simulink model "kinovaMicoSimscapeModel"  (R2021b)
settings: Solver=VariableStepAuto  StartTime=0.0  StopTime=0.3  FixedStep=0.01  RelTol=1e-3
PostLoadFcn:
  | micoRigidBodyTreeCreation;
  | IC=deg2rad([-90,180,180,0,0,0]);
  | interactiveHomePosition=deg2rad([-90 90 177.5 90 0 0]');
  | load("./KinovaMicoSimscapeVariantConfigurations.mat");
values from neighbouring files (symbols this model uses):
  micoCandlePosition = deg2rad([0,180,180,0,0,0])    [KinovaMicoSimscapeInitializeScript.m]    (also in generatingRandomTrajectory.m)
  ViaPointsTaskSpace = [ViaPointsTaskSpace;[[pi;0;pi],[pi;0;pi],[pi;0;pi],[pi;0;pi],[0;0;0],[0;0;0],[pi;0;pi]]]    [KinovaMicoSimscapeInitializeScript.m]    (also in generatingRandomTrajectory.m = [ViaPointsTaskSpace;zeros(3,7)])
undefined symbols (not defined in the file or in its folder): Mico, ViaPointsJointSpace, X, Y, Z
libraries: sm_lib x26, nesl_utility x19, robotcorelib x4, robotmaniplib x3, pid_lib x2
(part 29 of 50)

== matlab function kinovaMicoSimscapeModel/Variant Subsystem/TaskSpaceController/Adaptive PID/VectorManipulation ==
  data: dqr output; ddqr output; S output; q input; dq input; qd input; dqd input; ddqd input
function [dqr,ddqr,S] = VectorManipulation(q,dq,qd,dqd,ddqd)
%% Unpacking the measurements/desired points
%Unpackage the incoming reference/measured states

q1 = q(1);
q2 = q(2);
q3 = q(3);
q4 = q(4);
q5 = q(5);
q6 = q(6);

dq1 = dq(1);
dq2 = dq(2);
dq3 = dq(3);
dq4 = dq(4);
dq5 = dq(5);
dq6 = dq(6);

qd1 = qd(1);
qd2 = qd(2);
qd3 = qd(3);
qd4 = qd(4);
qd5 = qd(5);
qd6 = qd(6);

dqd1 = dqd(1);
dqd2 = dqd(2);
dqd3 = dqd(3);
dqd4 = dqd(4);
dqd5 = dqd(5);
dqd6 = dqd(6);

ddqd1 = ddqd(1);
ddqd2 = ddqd(2);
ddqd3 = ddqd(3);
ddqd4 = ddqd(4);
ddqd5 = ddqd(5);
ddqd6 = ddqd(6);

qError=q-qd;
dqError=dq-dqd;

%Define parameters
lambda=10*eye(6);
K=10;

dqr=dqd-lambda*qError;
ddqr=ddqd-lambda*dqError;

dqr1=dqr(1);
dqr2=dqr(2);
dqr3=dqr(3);
dqr4=dqr(4);
dqr5=dqr(5);
dqr6=dqr(6);

ddqr1=ddqr(1);
ddqr2=ddqr(2);
ddqr3=ddqr(3);
ddqr4=ddqr(4);
ddqr5=ddqr(5);
ddqr6=ddqr(6);

S=dqError+lambda*qError;

== matlab function kinovaMicoSimscapeModel/Variant Subsystem/TaskSpaceController/Enabled Subsystem/G_RNE ==
  data: q input; G output
function G = fcn(q)

q1 = q(1);
q2 = q(2);
q3 = q(3);
q4 = q(4);
q5 = q(5);
q6 = q(6);


G1 = 0;
 
G2 = (1116181*sin(q2))/2000000 + (41927301*cos(q2)*sin(q3))/200000000 - (41927301*cos(q3)*sin(q2))/200000000 + (164391*sin(q2)*sin(q3)*sin(q4))/5000000 + (164391*cos(q2)*cos(q3)*sin(q4))/5000000 + (213189*cos(q2)*cos(q5)*sin(q3))/200000000 - (213189*cos(q3)*cos(q5)*sin(q2))/200000000 + (3038029*3^(1/2)*cos(q2)*cos(q3)*sin(q4))/200000000 + (85507*3^(1/2)*cos(q2)*cos(q5)*sin(q3))/10000000 - (85507*3^(1/2)*cos(q3)*cos(q5)*sin(q2))/10000000 + (3038029*3^(1/2)*sin(q2)*sin(q3)*sin(q4))/200000000 - (85507*cos(q2)*cos(q3)*cos(q4)*sin(q5))/5000000 - (85507*cos(q2)*cos(q3)*cos(q5)*sin(q4))/10000000 - (85507*cos(q4)*sin(q2)*sin(q3)*sin(q5))/5000000 - (85507*cos(q5)*sin(q2)*sin(q3)*sin(q4))/10000000 - (71063*3^(1/2)*cos(q2)*cos(q3)*cos(q4)*sin(q5))/100000000 - (71063*3^(1/2)*cos(q2)*cos(q3)*cos(q5)*sin(q4))/200000000 - (71063*3^(1/2)*cos(q4)*sin(q2)*sin(q3)*sin(q5))/100000000 - (71063*3^(1/2)*cos(q5)*sin(q2)*sin(q3)*sin(q4))/200000000;
 
G3 = (41927301*cos(q3)*sin(q2))/200000000 - (41927301*cos(q2)*sin(q3))/200000000 - (164391*sin(q2)*sin(q3)*sin(q4))/5000000 - (164391*cos(q2)*cos(q3)*sin(q4))/5000000 - (213189*cos(q2)*cos(q5)*sin(q3))/200000000 + (213189*cos(q3)*cos(q5)*sin(q2))/200000000 - (3038029*3^(1/2)*cos(q2)*cos(q3)*sin(q4))/200000000 - (85507*3^(1/2)*cos(q2)*cos(q5)*sin(q3))/10000000 + (85507*3^(1/2)*cos(q3)*cos(q5)*sin(q2))/10000000 - (3038029*3^(1/2)*sin(q2)*sin(q3)*sin(q4))/200000000 + (85507*cos(q2)*cos(q3)*cos(q4)*sin(q5))/5000000 + (85507*cos(q2)*cos(q3)*cos(q5)*sin(q4))/10000000 + (85507*cos(q4)*sin(q2)*sin(q3)*sin(q5))/5000000 + (85507*cos(q5)*sin(q2)*sin(q3)*sin(q4))/10000000 + (71063*3^(1/2)*cos(q2)*cos(q3)*cos(q4)*sin(q5))/100000000 + (71063*3^(1/2)*cos(q2)*cos(q3)*cos(q5)*sin(q4))/200000000 + (71063*3^(1/2)*cos(q4)*sin(q2)*sin(q3)*sin(q5))/100000000 + (71063*3^(1/2)*cos(q5)*sin(q2)*sin(q3)*sin(q4))/200000000;
 
G4 = (164391*cos(q3)*cos(q4)*sin(q2))/5000000 - (164391*cos(q2)*cos(q4)*sin(q3))/5000000 - (3038029*3^(1/2)*cos(q2)*cos(q4)*sin(q3))/200000000 + (3038029*3^(1/2)*cos(q3)*cos(q4)*sin(q2))/200000000 + (85507*cos(q2)*cos(q4)*cos(q5)*sin(q3))/10000000 - (85507*cos(q3)*cos(q4)*cos(q5)*sin(q2))/10000000 - (85507*cos(q2)*sin(q3)*sin(q4)*sin(q5))/5000000 + (85507*cos(q3)*sin(q2)*sin(q4)*sin(q5))/5000000 + (71063*3^(1/2)*cos(q2)*cos(q4)*cos(q5)*sin(q3))/200000000 - (71063*3^(1/2)*cos(q3)*cos(q4)*cos(q5)*sin(q2))/200000000 - (71063*3^(1/2)*cos(q2)*sin(q3)*sin(q4)*sin(q5))/100000000 + (71063*3^(1/2)*cos(q3)*sin(q2)*sin(q4)*sin(q5))/100000000;
 
G5 = (85507*cos(q2)*cos(q4)*cos(q5)*sin(q3))/5000000 - (213189*cos(q2)*cos(q3)*sin(q5))/200000000 - (85507*3^(1/2)*cos(q2)*cos(q3)*sin(q5))/10000000 - (85507*3^(1/2)*sin(q2)*sin(q3)*sin(q5))/10000000 - (213189*sin(q2)*sin(q3)*sin(q5))/200000000 - (85507*cos(q3)*cos(q4)*cos(q5)*sin(q2))/5000000 - (85507*cos(q2)*sin(q3)*sin(q4)*sin(q5))/10000000 + (85507*cos(q3)*sin(q2)*sin(q4)*sin(q5))/10000000 + (71063*3^(1/2)*cos(q2)*cos(q4)*cos(q5)*sin(q3))/100000000 - (71063*3^(1/2)*cos(q3)*cos(q4)*cos(q5)*sin(q2))/100000000 - (71063*3^(1/2)*cos(q2)*sin(q3)*sin(q4)*sin(q5))/200000000 + (71063*3^(1/2)*cos(q3)*sin(q2)*sin(q4)*sin(q5))/200000000;
 
G6 = 0;
 
 
G =9.81.*[G1;
    G2;
    G3;
    G4;
    G5;
    G6];
